simulink model "ssc_lithium_cell_1RC_estim"  (Simulink 7.9)
settings: Solver=ode15s  StartTime=0  StopTime=37000  MaxStep=250  RelTol=1e-3
PreLoadFcn:
  | ssc_lithium_cell_1RC_estim_ini
undefined symbols (not defined in the file or in its folder): Capacity
libraries: LiBatteryElements_lib x4, nesl_utility x4, fl_lib x3
settings Model: Creator=psanghvi  LastModifiedBy=rjackey
settings DataIOCC: ExternalInput=[PulseData.time PulseData.current PulseData.voltage]  LimitDataPoints=off  LoadExternalInput=on  SignalLogging=off  DSMLogging=off
settings OptimizationCC: EnhancedBackFolding=on  OptimizeModelRefInitCode=on  LifeSpan=1  SimCompilerOptimization=On
settings DebuggingCC: FcnCallInpInsideContextMsg=Use local settings
settings RTWCC: SystemTargetFile=ert.tlc  GenCodeOnly=on  TemplateMakefile=ert_default_tmf  Description=Embedded Coder  GenerateReport=on  ProcessScript=ert_make_rtw_hook  IncludeHyperlinkInReport=on  LaunchReport=on  GenerateTraceInfo=on  GenerateTraceReport=on  GenerateTraceReportSl=on  GenerateTraceReportSf=on  GenerateTraceReportEml=on
settings CodeAppCC: IgnoreCustomStorageClasses=off
settings ERTTargetCC: CodeReplacementLibrary=ANSI_C  MultiwordLength=2048  GenerateSampleERTMain=on  ERTCustomFileTemplate=example_file_process.tlc  ConvertIfToSwitch=off  SuppressUnreachableDefaultCases=off

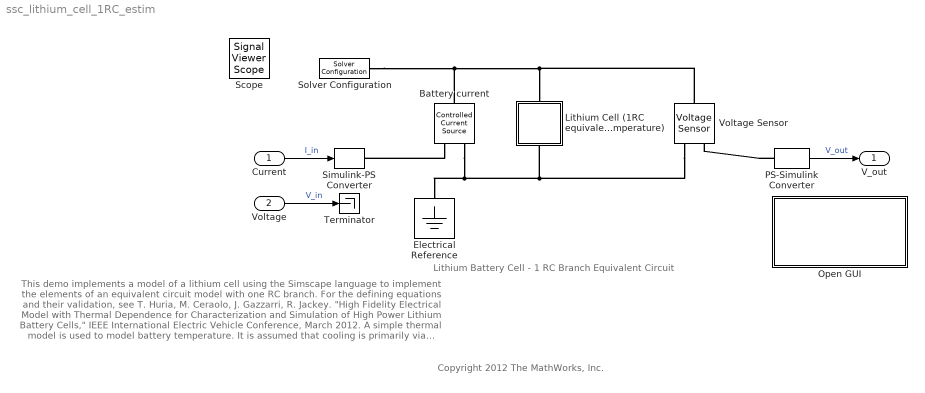
== system ssc_lithium_cell_1RC_estim ==
  note: Lithium Battery Cell - 1 RC Branch Equivalent Circuit
  note: This demo implements a model of a lithium cell using the Simscape language to implement the elements of an equivalent circuit model with one
      | RC branch. For the defining equations and their validation, see T. Huria, M. Ceraolo, J. Gazzarri, R. Jackey. "High Fidelity Electrical Model with
      | Thermal Dependence for Characterization and Simulation of High Power Lithium Battery Cells," IEEE International Electric Vehicle Conference,
      | March 2012. A simple thermal model is used to model battery temperature. It is assumed that cooling is primarily via convection, and that heating
      | is primarily from internal resistance. A battery pack can be modeled by connecting multiple copies of the battery cell block in series.
  note: Copyright 2012 The MathWorks, Inc.
  Current : Inport
  Voltage : Inport  Port=2
  Battery current : fl_lib/Electrical/Electrical Sources/Controlled Current Source  i_Log=off  v_Log=off  LocalVarNames=|current|voltage|power  LocalVarDescs=|Current (A)|Voltage (V)|Power (W)  LocalVarLogging=[0 0 0]
  Electrical Reference : fl_lib/Electrical/Electrical Elements/Electrical Reference  i_Log=off  LocalVarNames=|i  LocalVarDescs=|i  LocalVarLogging=[]
  "Lithium Cell (1RC equivalent circuit model,  single temperature)" : Subsystem
  Open GUI : Subsystem
      settings: OpenFcn=speload('ssc_lithium_cell_SDO_Project', 'Project - ssc_lithium_cell_1RC_estim', 'One Temp Estim');
      mask Display: disp('Double click here\nto open the\nParameter Estimation\nGUI with preloaded data')
  PS-Simulink Converter : nesl_utility/PS-Simulink Converter  PhysicalDomain=network_engine_domain  LeftPortType=input  RightPortType=output  SubClassName=ps_output  Unit=V  AffineConversion=off
  Simulink-PS Converter : nesl_utility/Simulink-PS Converter  PhysicalDomain=network_engine_domain  LeftPortType=input  RightPortType=output  SubClassName=ps_input  Unit=A  AffineConversion=off  InputFilterTimeConstant=.001  UdotUserProvided=0  SimscapeFilterOrder=1  InputFiltering=off
  Solver Configuration : nesl_utility/Solver Configuration  PhysicalDomain=network_engine_domain  LeftPortType=input  RightPortType=generic  SubClassName=solver  UseCustomDae=off  DoDC=off  ResidualTolerance=1e-9  UseLocalSolver=off  LocalSolverChoice=NE_BACKWARD_EULER_ADVANCER  LocalSolverSampleTime=.001  DoFixedCost=off  MaxNonlinIter=12  MaxModeIter=2  LinearAlgebra=Sparse  Accelerate=off  Profile=off  UseLocalSampling=off  DelaysMemoryBudget=1024
  Terminator : Terminator
  Voltage Sensor : fl_lib/Electrical/Electrical Sensors/Voltage Sensor  i1_Log=off  v1_Log=off  LocalVarNames=|i1|v1  LocalVarDescs=|i1|v1  LocalVarLogging=[]
  V_out : Outport
  Scope : SignalViewerScope  IOType=viewer  NumInputPorts=3  RefreshTime=0.035000
      settings: TimeRange=40000  YMin=3.15~-30~0  YMax=4.25~2~1
  wires:
  PS-Simulink Converter/1 -> V_out/1  "V_out"
  Current/1 -> Simulink-PS Converter/1  "I_in"
  Voltage/1 -> Terminator/1  "V_in"
  connections:
  Battery current/RConn1 -- Simulink-PS Converter/RConn1
  Battery current/LConn1 -- "Lithium Cell (1RC equivalent circuit model,  single temperature)"/LConn1 -- Voltage Sensor/LConn1 -- Solver Configuration/RConn1
  PS-Simulink Converter/LConn1 -- Voltage Sensor/RConn1
  Voltage Sensor/RConn2 -- "Lithium Cell (1RC equivalent circuit model,  single temperature)"/RConn1 -- Battery current/RConn2 -- Electrical Reference/LConn1

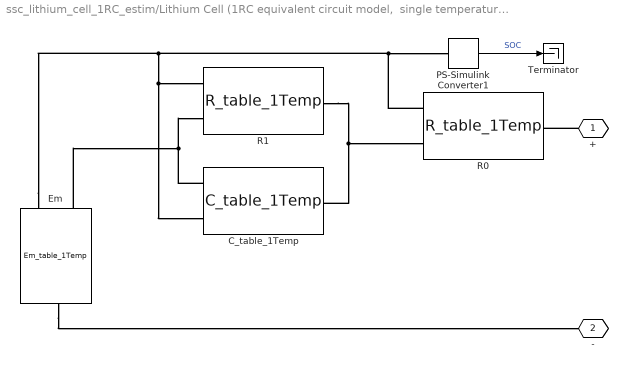
== system ssc_lithium_cell_1RC_estim/Lithium Cell (1RC equivalent circuit model,  single temperature) ==
  C_table_1Temp : LiBatteryElements_lib/C_table_1Temp  C_Table=C1 F  SOC_Table=SOC_LUT  v0=0 V  i_Log=off  v_Log=off  LocalVarNames=|i|v  LocalVarDescs=|i|v  LocalVarLogging=[0 0]
  Em : LiBatteryElements_lib/Em_table_1Temp  Em_Table=Em V  SOC_Table=SOC_LUT  C=Capacity hr*A  Qinit=Qe_init hr*A  i_Log=off  v_Log=off  Qe_Log=off  LocalVarNames=|i|v|Qe  LocalVarDescs=|i|v|Charge deficit  LocalVarLogging=[0 0 0]
  PS-Simulink Converter1 : nesl_utility/PS-Simulink Converter  PhysicalDomain=network_engine_domain  LeftPortType=input  RightPortType=output  SubClassName=ps_output  Unit=1  AffineConversion=off
  R0 : LiBatteryElements_lib/R_table_1Temp  R_Table=R0 Ohm  SOC_Table=SOC_LUT  i_Log=off  v_Log=off  LocalVarNames=|i|v  LocalVarDescs=|i|v  LocalVarLogging=[0 0]
  R1 : LiBatteryElements_lib/R_table_1Temp  R_Table=R1 Ohm  SOC_Table=SOC_LUT  i_Log=off  v_Log=off  LocalVarNames=|i|v  LocalVarDescs=|i|v  LocalVarLogging=[0 0]
  Terminator : Terminator
  + : PMIOPort  Tag=PMCPort  Port=1  Side=Left
  - : PMIOPort  Tag=PMCPort  Port=2  Side=Right
  wires:
  PS-Simulink Converter1/1 -> Terminator/1  "SOC"
  connections:
  Em/LConn1 -- C_table_1Temp/LConn1 -- R1/LConn1
  +/RConn1 -- R0/RConn1
  Em/RConn1 -- -/RConn1
  Em/LConn2 -- C_table_1Temp/LConn2 -- R1/LConn2 -- PS-Simulink Converter1/LConn1 -- R0/LConn2
  R1/RConn1 -- C_table_1Temp/RConn1 -- R0/LConn1

== system ssc_lithium_cell_1RC_estim/Open GUI ==
